simulink library "Analog"  (R2017a)
settings: Solver=VariableStepAuto  StartTime=0.0  StopTime=10.0  RelTol=1e-3
settings Model: Creator=Di Russo  LastModifiedBy=Vraj M

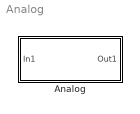
== system Analog ==
  Analog : Subsystem

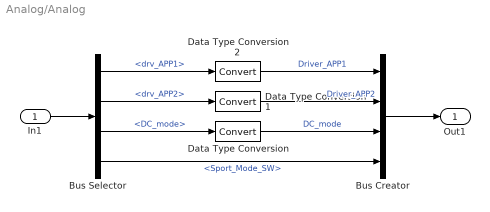
== system Analog/Analog ==
  In1 : Inport
  Bus Creator : BusCreator  Inputs=4
  Bus Selector : BusSelector  OutputSignals=Driver_Signals.drv_APP1,Driver_Signals.drv_APP2,DC_mode,Driver_Signals.Sport_Mode_SW
  Data Type Conversion : DataTypeConversion
  Data Type Conversion1 : DataTypeConversion
  Data Type Conversion2 : DataTypeConversion
  Out1 : Outport
  wires:
  Data Type Conversion/1 -> Bus Creator/3  "DC_mode"
  Data Type Conversion1/1 -> Bus Creator/2  "Driver_APP2"
  Data Type Conversion2/1 -> Bus Creator/1  "Driver_APP1"
  In1/1 -> Bus Selector/1
  Bus Creator/1 -> Out1/1
  Bus Selector/3 -> Data Type Conversion/1  "<DC_mode>"
  Bus Selector/2 -> Data Type Conversion1/1  "<drv_APP2>"
  Bus Selector/1 -> Data Type Conversion2/1  "<drv_APP1>"
  Bus Selector/4 -> Bus Creator/4  "<Sport_Mode_SW>"
